simulink model "spacecraft_assignment"  (R2024a)
settings: Solver=VariableStepAuto  StartTime=0.0  StopTime=50000  RelTol=1e-6  AbsTol=1e-6
model workspace (MAT data in the model file):
  q_initial = [0.7798 0.4125 0.4689 -0.0419]
  q_target = [0.1 0.2 0.3 0.2]
undefined symbols (not defined in the file or in its folder): IGRF
libraries: matrix_library x4, vrlib x3, eeGeneralControl x2, sharedtransform x2, aerolibanim x1
settings Model: Creator=vishwas  LastModifiedBy=vishwas
settings RTWCC: GPUComputeCapability=3.5

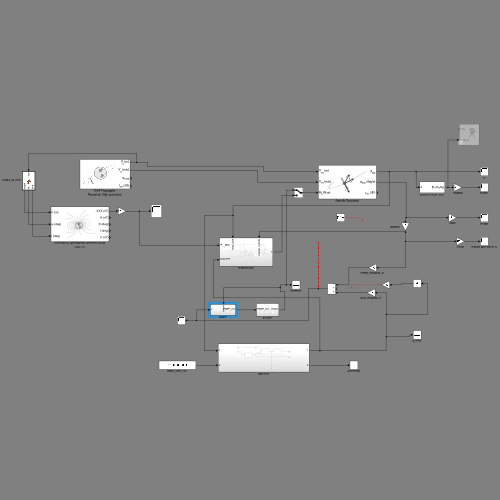
[thumbnail: Simulink's stored preview of the top-level diagram]
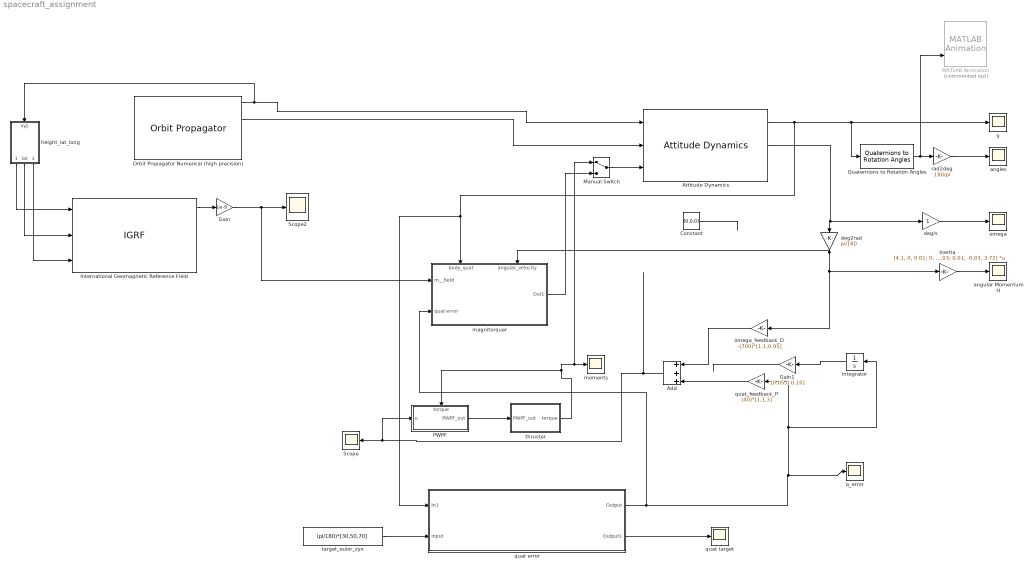
== system spacecraft_assignment ==
  Add : Sum  Inputs=+++
  Attitude Dynamics : AttitudeDynamics  mass=1  inertia=[4.1, 0, 0.01; 0, 4.3, -0.03; 0.01, -0.03, 3.72]  attitudeFrame=Fixed-frame  rotationOrder=ZYZ  attitudeRate=0*[15, -15, 15]
  Constant : Constant  Value=[0,0,0]
  Gain : Gain  Gain=1e-9
  Gain1 : Gain  Gain=[0.05,0.0,10]
  Inertia : Gain  Gain=[4.1, 0, 0.01; 0, 4.3, -0.03; 0.01, -0.03, 3.72]  Multiplication=Matrix(K*u)
  Integrator : Integrator
  International Geomagnetic Reference Field : IGRF  generation=IGRF-12  time_in=off  month=January  day=1  year=2020  sv_out=off
      settings: AttributesFormatString=%<generation>
  MATLAB Animation : aerolibanim/MATLAB Animation  Tag=Matlab Animation 6 DOF  Commented=on  Vehicles=1  Geometries='astredwedge.mat'  BoundingBoxCoordinates=[-50,50,-50,50,-50,50]  CameraOffset=[-150,-50,0]  CameraViewAngle=3  SampleTime=0.2  FigurePosition=[1983,1113,666,453]
  Manual Switch : ManualSwitch
  Orbit Propagator Numerical (high precision) : OrbitPropagator  propagator=Numerical (high precision)  outportFrame=Fixed-frame  semiMajorAxis=6971393  raan=30  argPeriapsis=90  trueAnomaly=10  inertialPosition=[3649700.0 3308200.0 -4676600.0]  inertialVelocity=[-2750.8 6666.4 2573.4]  fixedPosition=[-4142689.0 -2676864.7 -4669861.6]  fixedVelocity=[1452.7 -6720.7 2568.1]  gravityModel=Point-mass  customR=3396200  customMu=4.305e13  customJ2=1.0826269e-03  customOmega=4.06125949e-3  outputTransform=on  MagneticIndexExtrapMethod=IGRF  useOxygen=off
  PWPF : Subsystem
      settings: PortSchema="{\"entries\":[{\"content\":{\"sides\":[{\"content\":{\"connectorIds\":[\"In1\"]},\"type\":\"ConnectorPlacement.EquallySpacedRectSide\",\"uuid\":\"77e0a286-e0eb-42b2-9182-e4d488ef7559\"},{\"content\":{\"connectorIds\":[\"Out1\"],\"side\":\"RIGHT\"},\"type\":\"ConnectorPlacement.EquallySpacedRectSide\",\"uuid\":\"c1a301d0-2ccf-4655-ab50-bbc2e794ac88\"},{\"content\":{\"connectorIds\":[\"In2\"],\"side\":\"TOP\"},\"type\":\"ConnectorPlacement.EquallySpacedRectSide\",\"uuid\":\"a43bbc07-ff06-4e7a-a66b-73e4829b0f40\"}]},\"type\":\"ConnectorPlacement.EquallySpacedConnector\",\"uuid\":\"41bb159b-1b03-4419-9b29-11b1bd95012b\"}],\"packageUris\":[\"http://schema.mathworks.com/mf0/Connector/R2020b\"],\"version\":\"1.0\"}"
  Quaternions to Rotation Angles : sharedtransform/Quaternions to Rotation Angles  rotationOrder=ZYX  aMode=aMode
  Scope : Scope
  Scope2 : Scope
  angles : Scope
  angular Momentum H : Scope
  deg/s : Gain
  deg2rad : Gain  Gain=pi/180
  height_lat_long : MATLAB Function  TreatAsAtomicUnit=on
  magnitorquer : Subsystem
      settings: PortSchema="{\"entries\":[{\"content\":{\"sides\":[{\"content\":{\"connectorIds\":[\"In1\",\"In2\"]},\"type\":\"ConnectorPlacement.EquallySpacedRectSide\",\"uuid\":\"32674abe-99fc-4dff-8427-f22d1e0c988d\"},{\"content\":{\"connectorIds\":[\"Out1\"],\"side\":\"RIGHT\"},\"type\":\"ConnectorPlacement.EquallySpacedRectSide\",\"uuid\":\"a0511e2f-8dd2-4315-8603-e19834e52863\"},{\"content\":{\"connectorIds\":[\"In3\",\"In4\"],\"side\":\"TOP\"},\"type\":\"ConnectorPlacement.EquallySpacedRectSide\",\"uuid\":\"aa6fde77-ea81-4afc-b620-50aa6a1db330\"}]},\"type\":\"ConnectorPlacement.EquallySpacedConnector\",\"uuid\":\"f957fb2d-b253-46bf-a033-71b41e403e12\"}],\"packageUris\":[\"http://schema.mathworks.com/mf0/Connector/R2020b\"],\"version\":\"1.0\"}"
  moments : Scope
  omega : Scope
  omega_feedback_D : Gain  Gain=-(700)*[1,1,0.95]
  q : Scope
  q_error : Scope
  quat error : Subsystem
  quat target : Scope
  quat_feedback_P : Gain  Gain=(40)*[1,1,3]
  rad2deg : Gain  Gain=180/pi
  "target_euler_zyx " : Constant  Value=(pi/180)*[30,50,70]
  thruster : Subsystem
  wires:
  Orbit Propagator Numerical (high precision)/2 -> Attitude Dynamics/2
  omega_feedback_D/1 -> Add/1
  Quaternions to Rotation Angles/1 -> rad2deg/1, MATLAB Animation/2
  rad2deg/1 -> angles/1
  quat error/1(Output) -> magnitorquer/2(quat error), quat_feedback_P/1, Integrator/1, q_error/1
  quat error/2(Output1) -> quat target/1
  "target_euler_zyx "/1 -> quat error/2(Input)
  Inertia/1 -> angular Momentum H/1
  quat_feedback_P/1 -> Add/3
  Attitude Dynamics/2 -> deg2rad/1, deg/s/1
  Add/1 -> Scope/1, PWPF/1(u)
  deg2rad/1 -> Inertia/1, omega_feedback_D/1, magnitorquer/4(angular_velocity)
  height_lat_long/1(height) -> International Geomagnetic Reference Field/1
  height_lat_long/2(lat) -> International Geomagnetic Reference Field/2
  height_lat_long/3(long) -> International Geomagnetic Reference Field/3
  Attitude Dynamics/1 -> quat error/1(In1), magnitorquer/3(body_quat), q/1, Quaternions to Rotation Angles/1
  magnitorquer/1(Out1) -> Manual Switch/2
  Orbit Propagator Numerical (high precision)/1 -> Attitude Dynamics/1, height_lat_long/1(xyz)
  International Geomagnetic Reference Field/1 -> Gain/1
  Gain/1 -> magnitorquer/1(m__field), Scope2/1
  PWPF/1(PWPF_out) -> thruster/1(PWPF_out)
  Constant/1 -> ?
  Integrator/1 -> Gain1/1
  Gain1/1 -> ?
  deg/s/1 -> omega/1
  Manual Switch/1 -> Attitude Dynamics/3
  thruster/1(torque) -> PWPF/2(torque), Manual Switch/1, moments/1

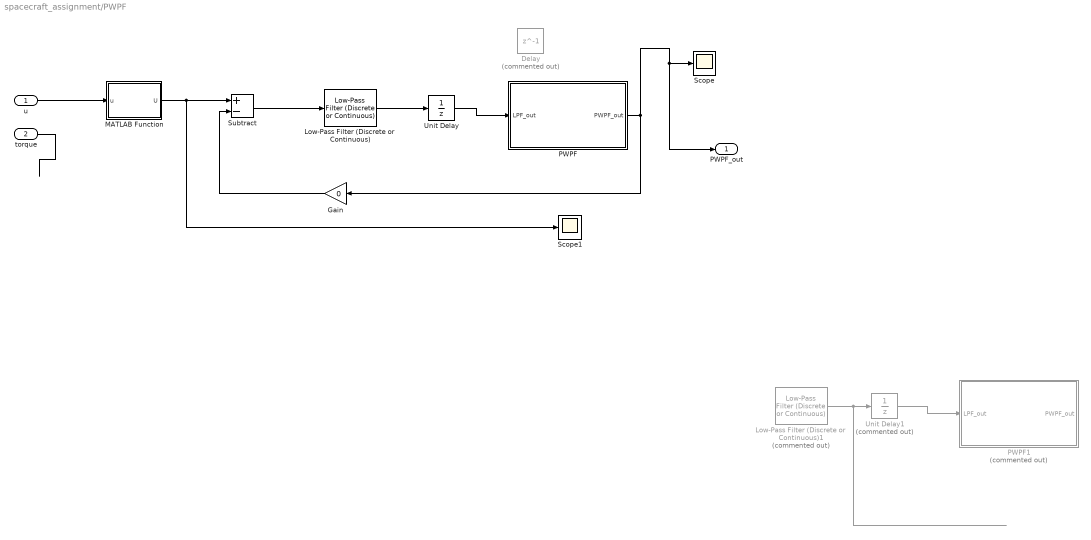
== system spacecraft_assignment/PWPF ==
  u : Inport
  torque : Inport  Port=2
  Delay : Delay  Commented=on  DelayLength=1  SampleTime=1
  Gain : Gain  Gain=0
  Low-Pass Filter (Discrete or Continuous) : eeGeneralControl/Low-Pass Filter (Discrete or Continuous)  K=10  T=0.128  B=inf  A=-inf  init_option=Inherited from block input  x0=0  Ts=-1
  Low-Pass Filter (Discrete or Continuous)1 : eeGeneralControl/Low-Pass Filter (Discrete or Continuous)  Commented=on  K=10  T=0.128  B=inf  A=-inf  init_option=Inherited from block input  x0=0  Ts=-1
  MATLAB Function : MATLAB Function  TreatAsAtomicUnit=on
  PWPF : MATLAB Function  TreatAsAtomicUnit=on
  PWPF1 : MATLAB Function  Commented=on  TreatAsAtomicUnit=on
  Scope : Scope
  Scope1 : Scope
  Subtract : Sum  Inputs=+-
  Unit Delay : UnitDelay  HasFrameUpgradeWarning=on
  Unit Delay1 : UnitDelay  Commented=on  HasFrameUpgradeWarning=on
  PWPF_out : Outport
  wires:
  u/1 -> MATLAB Function/1(u)
  PWPF/1(PWPF_out) -> Gain/1, PWPF_out/1, Scope/1
  Low-Pass Filter (Discrete or Continuous)/1 -> Unit Delay/1
  Subtract/1 -> Low-Pass Filter (Discrete or Continuous)/1
  Unit Delay/1 -> PWPF/1(LPF_out)
  Unit Delay1/1 -> PWPF1/1(LPF_out)
  Low-Pass Filter (Discrete or Continuous)1/1 -> Unit Delay1/1
  ? -> Low-Pass Filter (Discrete or Continuous)1/1
  MATLAB Function/1(U) -> Scope1/1, Subtract/1
  torque/1 -> ?
  Gain/1 -> Subtract/2

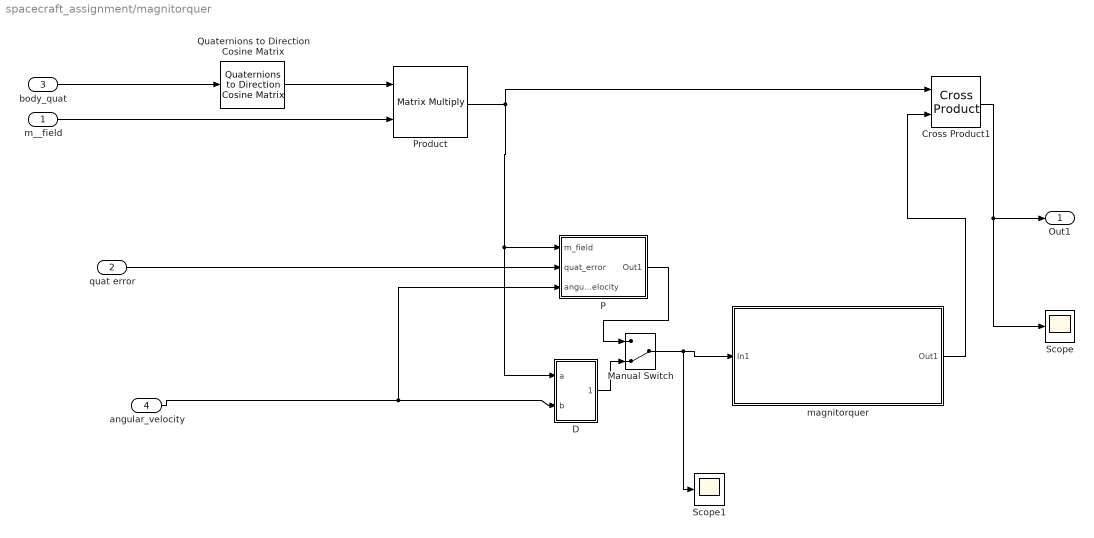
== system spacecraft_assignment/magnitorquer ==
  m__field : Inport
  quat error : Inport  Port=2
  body_quat : Inport  Port=3
  angular_velocity : Inport  Port=4
  Cross Product1 : matrix_library/Cross Product
  D : Subsystem
  Manual Switch : ManualSwitch  CurrentSetting=0
  P : Subsystem
  Product : Product  Multiplication=Matrix(*)
  Quaternions to Direction Cosine Matrix : sharedtransform/Quaternions to  Direction Cosine Matrix  aMode=aMode
      settings: LibrarySourceBlock=|
      | aerolibtransform2/Quaternions to
      | Direction Cosine Matrix
  Scope : Scope
  Scope1 : Scope
  magnitorquer : Subsystem
  Out1 : Outport
  wires:
  Product/1 -> D/1(a), P/1(m_field), Cross Product1/1
  body_quat/1 -> Quaternions to Direction Cosine Matrix/1
  magnitorquer/1(Out1) -> Cross Product1/2
  m__field/1 -> Product/2
  Quaternions to Direction Cosine Matrix/1 -> Product/1
  Cross Product1/1 -> Scope/1, Out1/1
  P/1(Out1) -> Manual Switch/1
  D/1(Out1) -> Manual Switch/2
  angular_velocity/1 -> P/3(angular_velocity), D/2(b)
  quat error/1 -> P/2(quat_error)
  Manual Switch/1 -> Scope1/1, magnitorquer/1(In1)

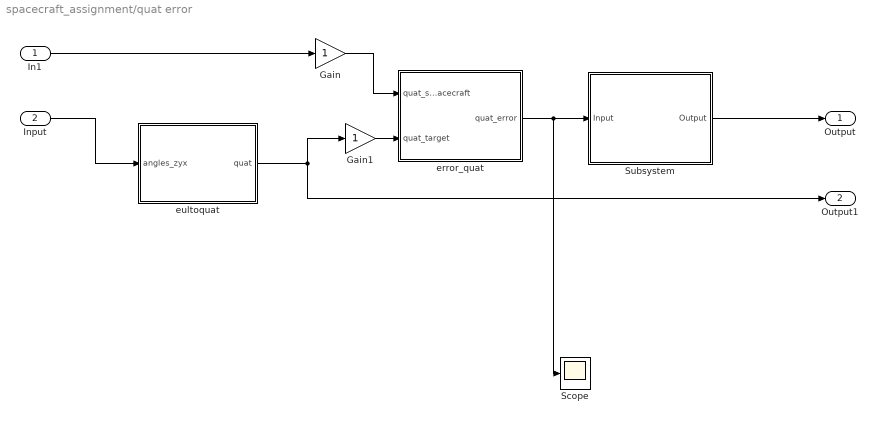
== system spacecraft_assignment/quat error ==
  In1 : Inport
  Input : Inport  Port=2
  Gain : Gain
  Gain1 : Gain
  Scope : Scope
  Subsystem : Subsystem
  "error_quat " : MATLAB Function  TreatAsAtomicUnit=on
  eultoquat : MATLAB Function  TreatAsAtomicUnit=on
  Output : Outport
  Output1 : Outport  Port=2
  wires:
  In1/1 -> Gain/1
  Subsystem/1(Output) -> Output/1
  eultoquat/1(quat) -> Gain1/1, Output1/1
  "error_quat "/1(quat_error) -> Scope/1, Subsystem/1(Input)
  Input/1 -> eultoquat/1(angles_zyx)
  Gain/1 -> "error_quat "/1(quat_spacecraft)
  Gain1/1 -> "error_quat "/2(quat_target)

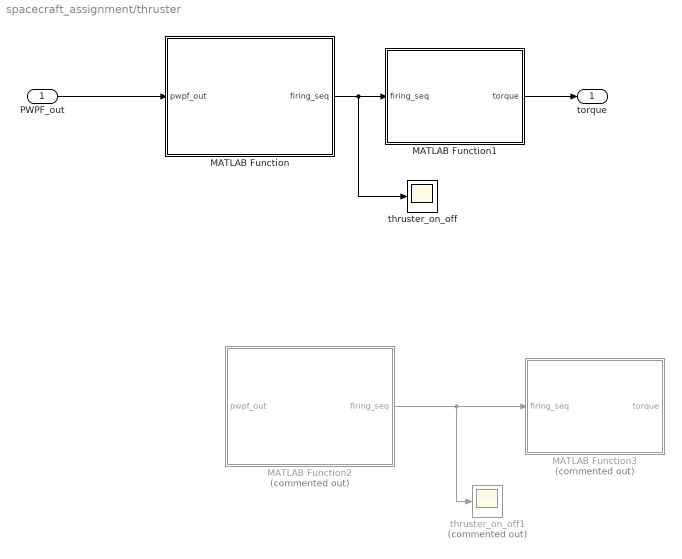
== system spacecraft_assignment/thruster ==
  PWPF_out : Inport
  MATLAB Function : MATLAB Function  TreatAsAtomicUnit=on
  MATLAB Function1 : MATLAB Function  TreatAsAtomicUnit=on
  MATLAB Function2 : MATLAB Function  Commented=on  TreatAsAtomicUnit=on
  MATLAB Function3 : MATLAB Function  Commented=on  TreatAsAtomicUnit=on
  thruster_on_off : Scope
      settings: Description=|
      | % to check which thruster is on
      | %none of the four thruster should have negative output
  thruster_on_off1 : Scope  Commented=on
      settings: Description=|
      | % to check which thruster is on
      | %none of the four thruster should have negative output
  torque : Outport
  wires:
  PWPF_out/1 -> MATLAB Function/1(pwpf_out)
  MATLAB Function/1(firing_seq) -> thruster_on_off/1, MATLAB Function1/1(firing_seq)
  MATLAB Function1/1(torque) -> torque/1
  MATLAB Function2/1(firing_seq) -> thruster_on_off1/1, MATLAB Function3/1(firing_seq)

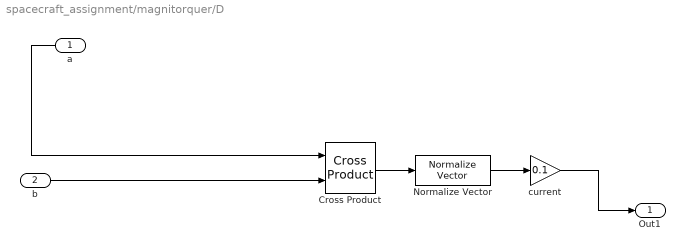
== system spacecraft_assignment/magnitorquer/D ==
  a : Inport
  b : Inport  Port=2
  Cross Product : matrix_library/Cross Product
  Normalize Vector : vrlib/Utilities/Normalize Vector  maxzero=0
  current : Gain  Gain=0.1
  Out1 : Outport
  wires:
  a/1 -> Cross Product/1
  current/1 -> Out1/1
  Normalize Vector/1 -> current/1
  b/1 -> Cross Product/2
  Cross Product/1 -> Normalize Vector/1

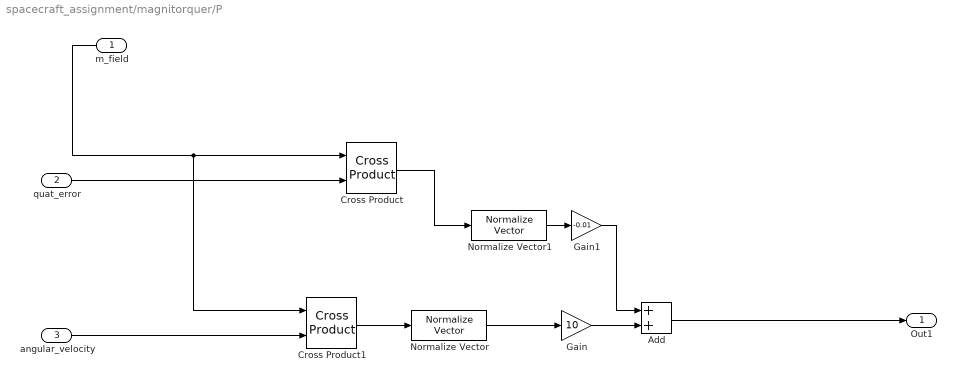
== system spacecraft_assignment/magnitorquer/P ==
  m_field : Inport
  quat_error : Inport  Port=2
  angular_velocity : Inport  Port=3
  Add : Sum
  Cross Product : matrix_library/Cross Product
  Cross Product1 : matrix_library/Cross Product
  Gain : Gain  Gain=10
  Gain1 : Gain  Gain=-0.01
  Normalize Vector : vrlib/Utilities/Normalize Vector  maxzero=0
  Normalize Vector1 : vrlib/Utilities/Normalize Vector  maxzero=0
  Out1 : Outport
  wires:
  Add/1 -> Out1/1
  m_field/1 -> Cross Product1/1, Cross Product/1
  quat_error/1 -> Cross Product/2
  Cross Product1/1 -> Normalize Vector/1
  angular_velocity/1 -> Cross Product1/2
  Cross Product/1 -> Normalize Vector1/1
  Gain/1 -> Add/2
  Normalize Vector1/1 -> Gain1/1
  Normalize Vector/1 -> Gain/1
  Gain1/1 -> Add/1

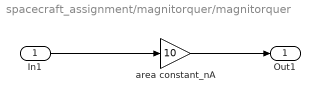
== system spacecraft_assignment/magnitorquer/magnitorquer ==
  In1 : Inport
  area constant_nA : Gain  Gain=10
  Out1 : Outport
  wires:
  In1/1 -> area constant_nA/1
  area constant_nA/1 -> Out1/1

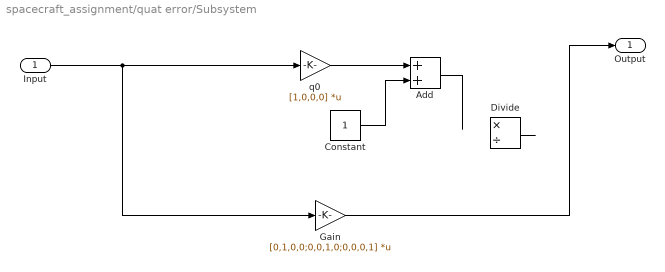
== system spacecraft_assignment/quat error/Subsystem ==
  Input : Inport  PortDimensions=4*1
  Add : Sum
  Constant : Constant
  Divide : Product  Inputs=*/
  Gain : Gain  Gain=[0,1,0,0;0,0,1,0;0,0,0,1]  Multiplication=Matrix(K*u)
  q0 : Gain  Gain=[1,0,0,0]  Multiplication=Matrix(K*u)
  Output : Outport
  wires:
  Input/1 -> q0/1, Gain/1
  Gain/1 -> Output/1
  q0/1 -> Add/1
  Constant/1 -> Add/2
  Add/1 -> ?
  Divide/1 -> ?

== matlab function spacecraft_assignment/quat error/error_quat  ==
  data: quat_spacecraft input; quat_error output; quat_target input
function quat_error = error_quat(quat_spacecraft,quat_target)

qs0 = quat_spacecraft(1);
qs1 = quat_spacecraft(2);
qs2 = quat_spacecraft(3);
qs3 = quat_spacecraft(4);


qt0 = quat_target(1);
qt1 = quat_target(2);
qt2 = quat_target(3);
qt3 = quat_target(4);


%quat 1 = world 2 body      
%quat 2 = world 2 target
%quat 3 = body 2 target == error

%quat2 = quat3*quat1;

%[TN]  = [TB][BN]

%need to figure out quat 3


%q = [P]*x
%x = [P]\q



Qs_mat=[qs0, -qs1, -qs2, -qs3;
        qs1,  qs0, -qs3,  qs2;
        qs2,  qs3,  qs0, -qs1;
        qs3, -qs2,  qs1,  qs0;];    %analytical mechanics of space systems pg 112




q = Qs_mat'*[qt0,qt1,qt2,qt3]';

%processing quat for error for 0/0 error when when tracking is achieved and
%track error is zero but numerically blows up due to inv(Qs_mat)



%
if q(1) < 0
    q = -q;
end


if abs(q(2)) <1e-10
    q(2) = 0;
end

if abs(q(3)) <1e-10
    q(3) = 0;
end

if abs(q(4)) < 1e-10
    q(4)=0;
end
%}

quat_error = q;

end

== matlab function spacecraft_assignment/height_lat_long ==
  data: height output; lat output; long output; xyz input
function [height,lat,long] = fcn(xyz)

 x = xyz(1);
 y = xyz(2);
 z = xyz(3);

 r = sqrt(x^2 + y^2 +z^2);
 R = 6371393;
 height = r-R;
 
 lat = asind(z/r);
 long = rad2deg(atan2(y,x));   % calculate lattitude and longitude 

 


end

== matlab function spacecraft_assignment/thruster/MATLAB Function2 ==
  data: pwpf_out input; firing_seq output
function firing_seq = thruster_selector(pwpf_out)

%total 4 thrusters
%each thruster has T thrust
%moment arm 150 mm from y and z axisfir

firing_seq = [0,0,0,0]';

tau_ideal = [ 0.0671   -0.0671    0.0671   -0.0671
             -0.1342         0    0.1342         0
                   0   -0.1342         0    0.1342];




p_M = pinv(tau_ideal);


time = p_M*pwpf_out;



for i = 1:4
    if abs(time(i)) < 1e-5
        time(i) = 0;
    end
end


for j = 1:4
    if sign(time(j)) == 1
        firing_seq(j) = 1;
    end
end




end

== matlab function spacecraft_assignment/PWPF/PWPF ==
  data: LPF_out input; PWPF_out output
function PWPF_out = PWPF_model(LPF_out)

    
    Um = 1;  

    Uon = 1;
    Uoff = 0.9;

    persistent PWPF_prev

    if isempty(PWPF_prev)
        PWPF_prev = [0,0,0]';
    end
    
    PWPF = PWPF_prev;
    

    for i = 1:3
        if (LPF_out(i,1) > Uon)
            PWPF(i,1) = Um;
            
        elseif (LPF_out(i,1) < -Uon)
            PWPF(i,1) = -Um;
            
        elseif (PWPF_prev(i,1) == 0)
            PWPF(i,1) = 0;
            
        elseif (PWPF_prev(i,1) > 0)
            if (LPF_out(i,1) < Uoff)
                PWPF(i,1) = 0;
            end

        elseif (LPF_out(i,1) > -Uoff)
            PWPF(i,1) = 0;
        end
    end



    PWPF_prev = PWPF;
    PWPF_out = PWPF;

end

== matlab function spacecraft_assignment/thruster/MATLAB Function ==
  data: pwpf_out input; firing_seq output
function firing_seq = thruster_selector(pwpf_out)

%total 4 thrusters
%each thruster has T thrust
%moment arm 150 mm from y and z axisfir
if norm(pwpf_out) == sqrt(3)
    pwpf_out = [1*pwpf_out(1),1*pwpf_out(2),1*pwpf_out(3)]';
end

firing_seq = logical([0,0,0,0]');

x = [pwpf_out(1);0;0];
y = [0;pwpf_out(2);0];
z = [0;0;pwpf_out(3)];

firing_seq_x = [1,1,1,1]';
firing_seq_y = [1,1,1,1]';
firing_seq_z = [1,1,1,1]';


%%
if pwpf_out(1) == 1
    firing_seq_x = [1,0,1,0]';
end

if pwpf_out(1) == -1
    firing_seq_x = [0,1,0,1]';
end


%%
if pwpf_out(2) == 1
    firing_seq_y = [0,1,1,1]';
end

if pwpf_out(2) == -1
    firing_seq_y = [1,1,0,1]';
end


%%
if pwpf_out(3) == 1
    firing_seq_z = [1,0,1,1]';
end

if pwpf_out(3) == -1
    firing_seq_z = [1,1,1,0]';
end

%%
if pwpf_out(1) == 0 && pwpf_out(2) == 0 && pwpf_out(3) == 0
    firing_seq_x = [0,0,0,0]';
    firing_seq_y = [0,0,0,0]';
    firing_seq_z = [0,0,0,0]';
end


firing_seq = firing_seq_x & firing_seq_y & firing_seq_z;



end

== matlab function spacecraft_assignment/thruster/MATLAB Function1 ==
  data: firing_seq input; torque output
function torque = body_torque(firing_seq)


T = 0.4;

T_vec = T*firing_seq;


tau_real = [ 0.0694   -0.0696    0.0643   -0.0640
            -0.1330    0.0070    0.1355   -0.0064
             0.0069   -0.1329   -0.0064    0.1357];

tau_ideal = [ 0.0671   -0.0671    0.0671   -0.0671
             -0.1342         0    0.1342         0
                   0   -0.1342         0    0.1342];


torque = tau_ideal*T_vec;

end

== matlab function spacecraft_assignment/thruster/MATLAB Function3 ==
  data: firing_seq input; torque output
function torque = body_torque(firing_seq)


T = 0.1;

T_vec = T*firing_seq;

tau_M = [ 0.0694   -0.0696    0.0643   -0.0640
         -0.1330    0.0070    0.1355   -0.0064
          0.0069   -0.1329   -0.0064    0.1357];

tau_ideal = [ 0.0671   -0.0671    0.0671   -0.0671
             -0.1342         0    0.1342         0
                   0   -0.1342         0    0.1342];


torque = tau_M*T_vec;

end

== matlab function spacecraft_assignment/PWPF/PWPF1 ==
  data: LPF_out input; PWPF_out output
function PWPF_out = PWPF_model(LPF_out)

    
    Um = 1;  

    Uon = 1;
    Uoff = -0.15;

    persistent PWPF_prev

    if isempty(PWPF_prev)
        PWPF_prev = [0,0,0]';
    end
    
    PWPF = PWPF_prev;
    

    for i = 1:3
        if (LPF_out(i,1) > Uon)
            PWPF(i,1) = Um;
            
        elseif (LPF_out(i,1) < -Uon)
            PWPF(i,1) = -Um;
            
        elseif (PWPF_prev(i,1) == 0)
            PWPF(i,1) = 0;
            
        elseif (PWPF_prev(i,1) > 0)
            if (LPF_out(i,1) < Uoff)
                PWPF(i,1) = 0;
            end

        elseif (LPF_out(i,1) > -Uoff)
            PWPF(i,1) = 0;
        end
    end



    PWPF_prev = PWPF;
    PWPF_out = PWPF;

end

== matlab function spacecraft_assignment/PWPF/MATLAB Function ==
  data: u input; U output
function U = fcn(u)

x = abs(u(1));
y = abs(u(2));
z = abs(u(3));

u1 = [x;y;z];

U = u;


min_u = min(u1);

for i = 1:3
    if abs(u(i)) == min_u
        U(i) = 0;
    end



end

== matlab function spacecraft_assignment/quat error/eultoquat ==
  data: angles_zyx input; quat output
function quat = fcn(angles_zyx)

quat = eul2quat([angles_zyx(1),angles_zyx(2),angles_zyx(3)],"ZYX");

end
